simulink model "task6_lab13"  (R2021a)
settings: Solver=VariableStepAuto  StartTime=0.0  StopTime=10.0  RelTol=1e-3
settings Model: Creator=reemb  LastModifiedBy=reemb

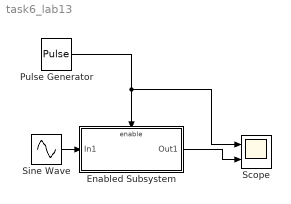
== system task6_lab13 ==
  Enabled Subsystem : Subsystem  TreatAsAtomicUnit=on
  Pulse Generator : DiscretePulseGenerator  Period=10  PulseWidth=5  SampleTime=0.125
  Scope : Scope  NumInputPorts=2
  Sine Wave : Sin  SampleTime=0
  wires:
  Pulse Generator/1 -> Scope/1, Enabled Subsystem/Enable
  Enabled Subsystem/1(Out1) -> Scope/2
  Sine Wave/1 -> Enabled Subsystem/1(In1)

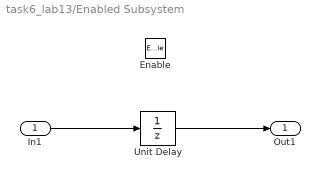
== system task6_lab13/Enabled Subsystem ==
  In1 : Inport
  Enable : EnablePort
  Unit Delay : UnitDelay  SampleTime=0.25  HasFrameUpgradeWarning=on
  Out1 : Outport
  wires:
  In1/1 -> Unit Delay/1
  Unit Delay/1 -> Out1/1
